simulink model "Array"
settings: Solver=VariableStepDiscrete  StartTime=0.0  StopTime=0.003  RelTol=1e-9  AbsTol=1e-9
values from neighbouring files (symbols this model uses):
  a11 = 300    [matlab1.mat]
  a12 = 200    [matlab1.mat]
  a13 = 100    [matlab1.mat]
  a14 = 100    [matlab1.mat]
  a15 = 100    [matlab1.mat]
  a16 = 100    [matlab1.mat]
  a21 = 200    [matlab1.mat]
  a22 = 100    [matlab1.mat]
  a23 = 100    [matlab1.mat]
  a24 = 1000    [matlab1.mat]
  a25 = 100    [matlab1.mat]
  a26 = 100    [matlab1.mat]
  a31 = 100    [matlab1.mat]
  a32 = 100    [matlab1.mat]
  a33 = 100    [matlab1.mat]
  a34 = 100    [matlab1.mat]
  a35 = 100    [matlab1.mat]
  a36 = 100    [matlab1.mat]
  a41 = 100    [matlab1.mat]
  a42 = 100    [matlab1.mat]
  a43 = 100    [matlab1.mat]
  a44 = 100    [matlab1.mat]
  a45 = 100    [matlab1.mat]
  a46 = 100    [matlab1.mat]
  a51 = 100    [matlab1.mat]
  a52 = 100    [matlab1.mat]
  a53 = 100    [matlab1.mat]
  a54 = 100    [matlab1.mat]
  a55 = 100    [matlab1.mat]
  a56 = 100    [matlab1.mat]
  a61 = 100    [matlab1.mat]
  a62 = 100    [matlab1.mat]
  a63 = 100    [matlab1.mat]
  a64 = 100    [matlab1.mat]
  a65 = 100    [matlab1.mat]
  a66 = 100    [matlab1.mat]
libraries: powerlib x154
(part 2 of 2)

== system Array/Array/PV panel35 ==
  Radiación : Inport
  Temperatura : Inport  Port=2
  Controlled Current Source : powerlib/Electrical Sources/Controlled Current Source  Initialize=on  Source_Type=AC  Amplitude=0  Phase=0  Frequency=0  Measurements=None
  Diode : powerlib/Power Electronics/Diode  Ron=0.001  Lon=0  Vf=0  IC=0  UseSnubber=off  Rs=500  Cs=250e-9  Measurements=off
  PV module : MATLAB Function  TreatAsAtomicUnit=on
  Vpv array : powerlib/Measurements/Voltage Measurement  PhasorSimulation=off  OutputType=Complex  PSBequivalent=0
  + : PMIOPort  Tag=PMCPort  Port=1  Side=Right
  - : PMIOPort  Tag=PMCPort  Port=2  Side=Right
  Ipv : Outport
  Vpv : Outport  Port=2
  wires:
  Radiación/1 -> PV module/2(Radiacion)
  Temperatura/1 -> PV module/3(Temp)
  PV module/1(I) -> Controlled Current Source/1, Ipv/1
  Vpv array/1 -> PV module/1(V), Vpv/1
  connections:
  Controlled Current Source/LConn1 -- Diode/LConn1 -- -/RConn1 -- Vpv array/LConn2
  Controlled Current Source/RConn1 -- Diode/RConn1 -- +/RConn1 -- Vpv array/LConn1

== system Array/Array/PV panel4 ==
  Radiación : Inport
  Temperatura : Inport  Port=2
  Controlled Current Source : powerlib/Electrical Sources/Controlled Current Source  Initialize=on  Source_Type=AC  Amplitude=0  Phase=0  Frequency=0  Measurements=None
  Diode : powerlib/Power Electronics/Diode  Ron=0.001  Lon=0  Vf=0  IC=0  UseSnubber=off  Rs=500  Cs=250e-9  Measurements=off
  PV module : MATLAB Function  TreatAsAtomicUnit=on
  Vpv array : powerlib/Measurements/Voltage Measurement  PhasorSimulation=off  OutputType=Complex  PSBequivalent=0
  + : PMIOPort  Tag=PMCPort  Port=1  Side=Right
  - : PMIOPort  Tag=PMCPort  Port=2  Side=Right
  Ipv : Outport
  Vpv : Outport  Port=2
  wires:
  Radiación/1 -> PV module/2(Radiacion)
  Temperatura/1 -> PV module/3(Temp)
  PV module/1(I) -> Controlled Current Source/1, Ipv/1
  Vpv array/1 -> PV module/1(V), Vpv/1
  connections:
  Controlled Current Source/LConn1 -- Diode/LConn1 -- -/RConn1 -- Vpv array/LConn2
  Controlled Current Source/RConn1 -- Diode/RConn1 -- +/RConn1 -- Vpv array/LConn1

== system Array/Array/PV panel5 ==
  Radiación : Inport
  Temperatura : Inport  Port=2
  Controlled Current Source : powerlib/Electrical Sources/Controlled Current Source  Initialize=on  Source_Type=AC  Amplitude=0  Phase=0  Frequency=0  Measurements=None
  Diode : powerlib/Power Electronics/Diode  Ron=0.001  Lon=0  Vf=0  IC=0  UseSnubber=off  Rs=500  Cs=250e-9  Measurements=off
  PV module : MATLAB Function  TreatAsAtomicUnit=on
  Vpv array : powerlib/Measurements/Voltage Measurement  PhasorSimulation=off  OutputType=Complex  PSBequivalent=0
  + : PMIOPort  Tag=PMCPort  Port=1  Side=Right
  - : PMIOPort  Tag=PMCPort  Port=2  Side=Right
  Ipv : Outport
  Vpv : Outport  Port=2
  wires:
  Radiación/1 -> PV module/2(Radiacion)
  Temperatura/1 -> PV module/3(Temp)
  PV module/1(I) -> Controlled Current Source/1, Ipv/1
  Vpv array/1 -> PV module/1(V), Vpv/1
  connections:
  Controlled Current Source/LConn1 -- Diode/LConn1 -- -/RConn1 -- Vpv array/LConn2
  Controlled Current Source/RConn1 -- Diode/RConn1 -- +/RConn1 -- Vpv array/LConn1

== system Array/Array/PV panel6 ==
  Radiación : Inport
  Temperatura : Inport  Port=2
  Controlled Current Source : powerlib/Electrical Sources/Controlled Current Source  Initialize=on  Source_Type=AC  Amplitude=0  Phase=0  Frequency=0  Measurements=None
  Diode : powerlib/Power Electronics/Diode  Ron=0.001  Lon=0  Vf=0  IC=0  UseSnubber=off  Rs=500  Cs=250e-9  Measurements=off
  PV module : MATLAB Function  TreatAsAtomicUnit=on
  Vpv array : powerlib/Measurements/Voltage Measurement  PhasorSimulation=off  OutputType=Complex  PSBequivalent=0
  + : PMIOPort  Tag=PMCPort  Port=1  Side=Right
  - : PMIOPort  Tag=PMCPort  Port=2  Side=Right
  Ipv : Outport
  Vpv : Outport  Port=2
  wires:
  Radiación/1 -> PV module/2(Radiacion)
  Temperatura/1 -> PV module/3(Temp)
  PV module/1(I) -> Controlled Current Source/1, Ipv/1
  Vpv array/1 -> PV module/1(V), Vpv/1
  connections:
  Controlled Current Source/LConn1 -- Diode/LConn1 -- -/RConn1 -- Vpv array/LConn2
  Controlled Current Source/RConn1 -- Diode/RConn1 -- +/RConn1 -- Vpv array/LConn1

== system Array/Array/PV panel7 ==
  Radiación : Inport
  Temperatura : Inport  Port=2
  Controlled Current Source : powerlib/Electrical Sources/Controlled Current Source  Initialize=on  Source_Type=AC  Amplitude=0  Phase=0  Frequency=0  Measurements=None
  Diode : powerlib/Power Electronics/Diode  Ron=0.001  Lon=0  Vf=0  IC=0  UseSnubber=off  Rs=500  Cs=250e-9  Measurements=off
  PV module : MATLAB Function  TreatAsAtomicUnit=on
  Vpv array : powerlib/Measurements/Voltage Measurement  PhasorSimulation=off  OutputType=Complex  PSBequivalent=0
  + : PMIOPort  Tag=PMCPort  Port=1  Side=Right
  - : PMIOPort  Tag=PMCPort  Port=2  Side=Right
  Ipv : Outport
  Vpv : Outport  Port=2
  wires:
  Radiación/1 -> PV module/2(Radiacion)
  Temperatura/1 -> PV module/3(Temp)
  PV module/1(I) -> Controlled Current Source/1, Ipv/1
  Vpv array/1 -> PV module/1(V), Vpv/1
  connections:
  Controlled Current Source/LConn1 -- Diode/LConn1 -- -/RConn1 -- Vpv array/LConn2
  Controlled Current Source/RConn1 -- Diode/RConn1 -- +/RConn1 -- Vpv array/LConn1

== system Array/Array/PV panel8 ==
  Radiación : Inport
  Temperatura : Inport  Port=2
  Controlled Current Source : powerlib/Electrical Sources/Controlled Current Source  Initialize=on  Source_Type=AC  Amplitude=0  Phase=0  Frequency=0  Measurements=None
  Diode : powerlib/Power Electronics/Diode  Ron=0.001  Lon=0  Vf=0  IC=0  UseSnubber=off  Rs=500  Cs=250e-9  Measurements=off
  PV module : MATLAB Function  TreatAsAtomicUnit=on
  Vpv array : powerlib/Measurements/Voltage Measurement  PhasorSimulation=off  OutputType=Complex  PSBequivalent=0
  + : PMIOPort  Tag=PMCPort  Port=1  Side=Right
  - : PMIOPort  Tag=PMCPort  Port=2  Side=Right
  Ipv : Outport
  Vpv : Outport  Port=2
  wires:
  Radiación/1 -> PV module/2(Radiacion)
  Temperatura/1 -> PV module/3(Temp)
  PV module/1(I) -> Controlled Current Source/1, Ipv/1
  Vpv array/1 -> PV module/1(V), Vpv/1
  connections:
  Controlled Current Source/LConn1 -- Diode/LConn1 -- -/RConn1 -- Vpv array/LConn2
  Controlled Current Source/RConn1 -- Diode/RConn1 -- +/RConn1 -- Vpv array/LConn1

== system Array/Array/PV panel9 ==
  Radiación : Inport
  Temperatura : Inport  Port=2
  Controlled Current Source : powerlib/Electrical Sources/Controlled Current Source  Initialize=on  Source_Type=AC  Amplitude=0  Phase=0  Frequency=0  Measurements=None
  Diode : powerlib/Power Electronics/Diode  Ron=0.001  Lon=0  Vf=0  IC=0  UseSnubber=off  Rs=500  Cs=250e-9  Measurements=off
  PV module : MATLAB Function  TreatAsAtomicUnit=on
  Vpv array : powerlib/Measurements/Voltage Measurement  PhasorSimulation=off  OutputType=Complex  PSBequivalent=0
  + : PMIOPort  Tag=PMCPort  Port=1  Side=Right
  - : PMIOPort  Tag=PMCPort  Port=2  Side=Right
  Ipv : Outport
  Vpv : Outport  Port=2
  wires:
  Radiación/1 -> PV module/2(Radiacion)
  Temperatura/1 -> PV module/3(Temp)
  PV module/1(I) -> Controlled Current Source/1, Ipv/1
  Vpv array/1 -> PV module/1(V), Vpv/1
  connections:
  Controlled Current Source/LConn1 -- Diode/LConn1 -- -/RConn1 -- Vpv array/LConn2
  Controlled Current Source/RConn1 -- Diode/RConn1 -- +/RConn1 -- Vpv array/LConn1

== matlab function Array/PV panel1/PV module ==
  data: V input; I output; Radiacion input; Temp input
function I = Panel (V,Radiacion,Temp)
% Carga del Electron
q=1.602176e-19;
% Contante de Boltzman
K=1.3806488e-23;
% Constante del material
n=1.3;
% Temperatura en Kelvin
T=273.15+Temp;
% Resistencia serie
Rs=0.015;
% Resistencia Paralelo
Rp=100;
% Calculo del producto de constantes de la exponencial
Vt=(n*K*T)/q;
Ns=36; %celdas en serie.
Vc=V./Ns;
% Corriente de Fotogenerada
Isc=5.433;
Alfa=0.037/100;
%variacion de la corriente con la temperatura
Iph=Isc*Radiacion/1000*(1+(Alfa*(Temp-25)));
% Corriente inversa del diodo
Voc_ref=22.2/Ns;
Beta=-0.34/100;
Voc=Voc_ref*(1+(Beta*(Temp-25)));
%for i=1:length(Vc)
%if (Vc(i)>Voc)
%Vc(i)=Voc;
%end
%end
Io=Isc/(exp(Voc/Vt)-1);
Ir=Io;%*(T/298.15)^3*exp(((T/298.15)-1)*1.11*q/(n*K*298.15));

% Funcion a Valuar
I=zeros(size(Vc));
for i=1:50
I = I - (Iph - I - Ir .* ( exp((Vc + I .* Rs) ./ Vt) -1)+(Vc + I .* Rs)/Rp)... 
        ./ (-1 - Ir * (Rs ./ Vt) .* exp((Vc + I .* Rs) ./ Vt)-Rs/Rp); 
end
 end

== matlab function Array/PV panel/PV module ==
  data: V input; I output; Radiacion input; Temp input
function I = Panel (V,Radiacion,Temp)
% Carga del Electron
q=1.602176e-19;
% Contante de Boltzman
K=1.3806488e-23;
% Constante del material
n=1.3;
% Temperatura en Kelvin
T=273.15+Temp;
% Resistencia serie
Rs=0.015;
% Resistencia Paralelo
Rp=100;
% Calculo del producto de constantes de la exponencial
Vt=(n*K*T)/q;
Ns=36; %celdas en serie.
Vc=V./Ns;
% Corriente de Fotogenerada
Isc=5.433;
Alfa=0.037/100;
%variacion de la corriente con la temperatura
Iph=Isc*Radiacion/1000*(1+(Alfa*(Temp-25)));
% Corriente inversa del diodo
Voc_ref=22.2/Ns;
Beta=-0.34/100;
Voc=Voc_ref*(1+(Beta*(Temp-25)));
%for i=1:length(Vc)
%if (Vc(i)>Voc)
%Vc(i)=Voc;
%end
%end
Io=Isc/(exp(Voc/Vt)-1);
Ir=Io;%*(T/298.15)^3*exp(((T/298.15)-1)*1.11*q/(n*K*298.15));

% Funcion a Valuar
I=zeros(size(Vc));
for i=1:50
I = I - (Iph - I - Ir .* ( exp((Vc + I .* Rs) ./ Vt) -1)+(Vc + I .* Rs)/Rp)... 
        ./ (-1 - Ir * (Rs ./ Vt) .* exp((Vc + I .* Rs) ./ Vt)-Rs/Rp); 
end
 end

== matlab function Array/PV panel2/PV module ==
  data: V input; I output; Radiacion input; Temp input
function I = Panel (V,Radiacion,Temp)
% Carga del Electron
q=1.602176e-19;
% Contante de Boltzman
K=1.3806488e-23;
% Constante del material
n=1.3;
% Temperatura en Kelvin
T=273.15+Temp;
% Resistencia serie
Rs=0.015;
% Resistencia Paralelo
Rp=100;
% Calculo del producto de constantes de la exponencial
Vt=(n*K*T)/q;
Ns=36; %celdas en serie.
Vc=V./Ns;
% Corriente de Fotogenerada
Isc=5.433;
Alfa=0.037/100;
%variacion de la corriente con la temperatura
Iph=Isc*Radiacion/1000*(1+(Alfa*(Temp-25)));
% Corriente inversa del diodo
Voc_ref=22.2/Ns;
Beta=-0.34/100;
Voc=Voc_ref*(1+(Beta*(Temp-25)));
%for i=1:length(Vc)
%if (Vc(i)>Voc)
%Vc(i)=Voc;
%end
%end
Io=Isc/(exp(Voc/Vt)-1);
Ir=Io;%*(T/298.15)^3*exp(((T/298.15)-1)*1.11*q/(n*K*298.15));

% Funcion a Valuar
I=zeros(size(Vc));
for i=1:50
I = I - (Iph - I - Ir .* ( exp((Vc + I .* Rs) ./ Vt) -1)+(Vc + I .* Rs)/Rp)... 
        ./ (-1 - Ir * (Rs ./ Vt) .* exp((Vc + I .* Rs) ./ Vt)-Rs/Rp); 
end
 end

== matlab function Array/PV panel3/PV module ==
  data: V input; I output; Radiacion input; Temp input
function I = Panel (V,Radiacion,Temp)
% Carga del Electron
q=1.602176e-19;
% Contante de Boltzman
K=1.3806488e-23;
% Constante del material
n=1.3;
% Temperatura en Kelvin
T=273.15+Temp;
% Resistencia serie
Rs=0.015;
% Resistencia Paralelo
Rp=100;
% Calculo del producto de constantes de la exponencial
Vt=(n*K*T)/q;
Ns=36; %celdas en serie.
Vc=V./Ns;
% Corriente de Fotogenerada
Isc=5.433;
Alfa=0.037/100;
%variacion de la corriente con la temperatura
Iph=Isc*Radiacion/1000*(1+(Alfa*(Temp-25)));
% Corriente inversa del diodo
Voc_ref=22.2/Ns;
Beta=-0.34/100;
Voc=Voc_ref*(1+(Beta*(Temp-25)));
%for i=1:length(Vc)
%if (Vc(i)>Voc)
%Vc(i)=Voc;
%end
%end
Io=Isc/(exp(Voc/Vt)-1);
Ir=Io;%*(T/298.15)^3*exp(((T/298.15)-1)*1.11*q/(n*K*298.15));

% Funcion a Valuar
I=zeros(size(Vc));
for i=1:50
I = I - (Iph - I - Ir .* ( exp((Vc + I .* Rs) ./ Vt) -1)+(Vc + I .* Rs)/Rp)... 
        ./ (-1 - Ir * (Rs ./ Vt) .* exp((Vc + I .* Rs) ./ Vt)-Rs/Rp); 
end
 end

== matlab function Array/PV panel4/PV module ==
  data: V input; I output; Radiacion input; Temp input
function I = Panel (V,Radiacion,Temp)
% Carga del Electron
q=1.602176e-19;
% Contante de Boltzman
K=1.3806488e-23;
% Constante del material
n=1.3;
% Temperatura en Kelvin
T=273.15+Temp;
% Resistencia serie
Rs=0.015;
% Resistencia Paralelo
Rp=100;
% Calculo del producto de constantes de la exponencial
Vt=(n*K*T)/q;
Ns=36; %celdas en serie.
Vc=V./Ns;
% Corriente de Fotogenerada
Isc=5.433;
Alfa=0.037/100;
%variacion de la corriente con la temperatura
Iph=Isc*Radiacion/1000*(1+(Alfa*(Temp-25)));
% Corriente inversa del diodo
Voc_ref=22.2/Ns;
Beta=-0.34/100;
Voc=Voc_ref*(1+(Beta*(Temp-25)));
%for i=1:length(Vc)
%if (Vc(i)>Voc)
%Vc(i)=Voc;
%end
%end
Io=Isc/(exp(Voc/Vt)-1);
Ir=Io;%*(T/298.15)^3*exp(((T/298.15)-1)*1.11*q/(n*K*298.15));

% Funcion a Valuar
I=zeros(size(Vc));
for i=1:50
I = I - (Iph - I - Ir .* ( exp((Vc + I .* Rs) ./ Vt) -1)+(Vc + I .* Rs)/Rp)... 
        ./ (-1 - Ir * (Rs ./ Vt) .* exp((Vc + I .* Rs) ./ Vt)-Rs/Rp); 
end
 end

== matlab function Array/PV panel5/PV module ==
  data: V input; I output; Radiacion input; Temp input
function I = Panel (V,Radiacion,Temp)
% Carga del Electron
q=1.602176e-19;
% Contante de Boltzman
K=1.3806488e-23;
% Constante del material
n=1.3;
% Temperatura en Kelvin
T=273.15+Temp;
% Resistencia serie
Rs=0.015;
% Resistencia Paralelo
Rp=100;
% Calculo del producto de constantes de la exponencial
Vt=(n*K*T)/q;
Ns=36; %celdas en serie.
Vc=V./Ns;
% Corriente de Fotogenerada
Isc=5.433;
Alfa=0.037/100;
%variacion de la corriente con la temperatura
Iph=Isc*Radiacion/1000*(1+(Alfa*(Temp-25)));
% Corriente inversa del diodo
Voc_ref=22.2/Ns;
Beta=-0.34/100;
Voc=Voc_ref*(1+(Beta*(Temp-25)));
%for i=1:length(Vc)
%if (Vc(i)>Voc)
%Vc(i)=Voc;
%end
%end
Io=Isc/(exp(Voc/Vt)-1);
Ir=Io;%*(T/298.15)^3*exp(((T/298.15)-1)*1.11*q/(n*K*298.15));

% Funcion a Valuar
I=zeros(size(Vc));
for i=1:50
I = I - (Iph - I - Ir .* ( exp((Vc + I .* Rs) ./ Vt) -1)+(Vc + I .* Rs)/Rp)... 
        ./ (-1 - Ir * (Rs ./ Vt) .* exp((Vc + I .* Rs) ./ Vt)-Rs/Rp); 
end
 end

== matlab function Array/PV panel6/PV module ==
  data: V input; I output; Radiacion input; Temp input
function I = Panel (V,Radiacion,Temp)
% Carga del Electron
q=1.602176e-19;
% Contante de Boltzman
K=1.3806488e-23;
% Constante del material
n=1.3;
% Temperatura en Kelvin
T=273.15+Temp;
% Resistencia serie
Rs=0.015;
% Resistencia Paralelo
Rp=100;
% Calculo del producto de constantes de la exponencial
Vt=(n*K*T)/q;
Ns=36; %celdas en serie.
Vc=V./Ns;
% Corriente de Fotogenerada
Isc=5.433;
Alfa=0.037/100;
%variacion de la corriente con la temperatura
Iph=Isc*Radiacion/1000*(1+(Alfa*(Temp-25)));
% Corriente inversa del diodo
Voc_ref=22.2/Ns;
Beta=-0.34/100;
Voc=Voc_ref*(1+(Beta*(Temp-25)));
%for i=1:length(Vc)
%if (Vc(i)>Voc)
%Vc(i)=Voc;
%end
%end
Io=Isc/(exp(Voc/Vt)-1);
Ir=Io;%*(T/298.15)^3*exp(((T/298.15)-1)*1.11*q/(n*K*298.15));

% Funcion a Valuar
I=zeros(size(Vc));
for i=1:50
I = I - (Iph - I - Ir .* ( exp((Vc + I .* Rs) ./ Vt) -1)+(Vc + I .* Rs)/Rp)... 
        ./ (-1 - Ir * (Rs ./ Vt) .* exp((Vc + I .* Rs) ./ Vt)-Rs/Rp); 
end
 end

== matlab function Array/PV panel7/PV module ==
  data: V input; I output; Radiacion input; Temp input
function I = Panel (V,Radiacion,Temp)
% Carga del Electron
q=1.602176e-19;
% Contante de Boltzman
K=1.3806488e-23;
% Constante del material
n=1.3;
% Temperatura en Kelvin
T=273.15+Temp;
% Resistencia serie
Rs=0.015;
% Resistencia Paralelo
Rp=100;
% Calculo del producto de constantes de la exponencial
Vt=(n*K*T)/q;
Ns=36; %celdas en serie.
Vc=V./Ns;
% Corriente de Fotogenerada
Isc=5.433;
Alfa=0.037/100;
%variacion de la corriente con la temperatura
Iph=Isc*Radiacion/1000*(1+(Alfa*(Temp-25)));
% Corriente inversa del diodo
Voc_ref=22.2/Ns;
Beta=-0.34/100;
Voc=Voc_ref*(1+(Beta*(Temp-25)));
%for i=1:length(Vc)
%if (Vc(i)>Voc)
%Vc(i)=Voc;
%end
%end
Io=Isc/(exp(Voc/Vt)-1);
Ir=Io;%*(T/298.15)^3*exp(((T/298.15)-1)*1.11*q/(n*K*298.15));

% Funcion a Valuar
I=zeros(size(Vc));
for i=1:50
I = I - (Iph - I - Ir .* ( exp((Vc + I .* Rs) ./ Vt) -1)+(Vc + I .* Rs)/Rp)... 
        ./ (-1 - Ir * (Rs ./ Vt) .* exp((Vc + I .* Rs) ./ Vt)-Rs/Rp); 
end
 end

== matlab function Array/PV panel8/PV module ==
  data: V input; I output; Radiacion input; Temp input
function I = Panel (V,Radiacion,Temp)
% Carga del Electron
q=1.602176e-19;
% Contante de Boltzman
K=1.3806488e-23;
% Constante del material
n=1.3;
% Temperatura en Kelvin
T=273.15+Temp;
% Resistencia serie
Rs=0.015;
% Resistencia Paralelo
Rp=100;
% Calculo del producto de constantes de la exponencial
Vt=(n*K*T)/q;
Ns=36; %celdas en serie.
Vc=V./Ns;
% Corriente de Fotogenerada
Isc=5.433;
Alfa=0.037/100;
%variacion de la corriente con la temperatura
Iph=Isc*Radiacion/1000*(1+(Alfa*(Temp-25)));
% Corriente inversa del diodo
Voc_ref=22.2/Ns;
Beta=-0.34/100;
Voc=Voc_ref*(1+(Beta*(Temp-25)));
%for i=1:length(Vc)
%if (Vc(i)>Voc)
%Vc(i)=Voc;
%end
%end
Io=Isc/(exp(Voc/Vt)-1);
Ir=Io;%*(T/298.15)^3*exp(((T/298.15)-1)*1.11*q/(n*K*298.15));

% Funcion a Valuar
I=zeros(size(Vc));
for i=1:50
I = I - (Iph - I - Ir .* ( exp((Vc + I .* Rs) ./ Vt) -1)+(Vc + I .* Rs)/Rp)... 
        ./ (-1 - Ir * (Rs ./ Vt) .* exp((Vc + I .* Rs) ./ Vt)-Rs/Rp); 
end
 end

== matlab function Array/PV panel10/PV module ==
  data: V input; I output; Radiacion input; Temp input
function I = Panel (V,Radiacion,Temp)
% Carga del Electron
q=1.602176e-19;
% Contante de Boltzman
K=1.3806488e-23;
% Constante del material
n=1.3;
% Temperatura en Kelvin
T=273.15+Temp;
% Resistencia serie
Rs=0.015;
% Resistencia Paralelo
Rp=100;
% Calculo del producto de constantes de la exponencial
Vt=(n*K*T)/q;
Ns=36; %celdas en serie.
Vc=V./Ns;
% Corriente de Fotogenerada
Isc=5.433;
Alfa=0.037/100;
%variacion de la corriente con la temperatura
Iph=Isc*Radiacion/1000*(1+(Alfa*(Temp-25)));
% Corriente inversa del diodo
Voc_ref=22.2/Ns;
Beta=-0.34/100;
Voc=Voc_ref*(1+(Beta*(Temp-25)));
%for i=1:length(Vc)
%if (Vc(i)>Voc)
%Vc(i)=Voc;
%end
%end
Io=Isc/(exp(Voc/Vt)-1);
Ir=Io;%*(T/298.15)^3*exp(((T/298.15)-1)*1.11*q/(n*K*298.15));

% Funcion a Valuar
I=zeros(size(Vc));
for i=1:50
I = I - (Iph - I - Ir .* ( exp((Vc + I .* Rs) ./ Vt) -1)+(Vc + I .* Rs)/Rp)... 
        ./ (-1 - Ir * (Rs ./ Vt) .* exp((Vc + I .* Rs) ./ Vt)-Rs/Rp); 
end
 end

== matlab function Array/PV panel11/PV module ==
  data: V input; I output; Radiacion input; Temp input
function I = Panel (V,Radiacion,Temp)
% Carga del Electron
q=1.602176e-19;
% Contante de Boltzman
K=1.3806488e-23;
% Constante del material
n=1.3;
% Temperatura en Kelvin
T=273.15+Temp;
% Resistencia serie
Rs=0.015;
% Resistencia Paralelo
Rp=100;
% Calculo del producto de constantes de la exponencial
Vt=(n*K*T)/q;
Ns=36; %celdas en serie.
Vc=V./Ns;
% Corriente de Fotogenerada
Isc=5.433;
Alfa=0.037/100;
%variacion de la corriente con la temperatura
Iph=Isc*Radiacion/1000*(1+(Alfa*(Temp-25)));
% Corriente inversa del diodo
Voc_ref=22.2/Ns;
Beta=-0.34/100;
Voc=Voc_ref*(1+(Beta*(Temp-25)));
%for i=1:length(Vc)
%if (Vc(i)>Voc)
%Vc(i)=Voc;
%end
%end
Io=Isc/(exp(Voc/Vt)-1);
Ir=Io;%*(T/298.15)^3*exp(((T/298.15)-1)*1.11*q/(n*K*298.15));

% Funcion a Valuar
I=zeros(size(Vc));
for i=1:50
I = I - (Iph - I - Ir .* ( exp((Vc + I .* Rs) ./ Vt) -1)+(Vc + I .* Rs)/Rp)... 
        ./ (-1 - Ir * (Rs ./ Vt) .* exp((Vc + I .* Rs) ./ Vt)-Rs/Rp); 
end
 end

== matlab function Array/PV panel12/PV module ==
  data: V input; I output; Radiacion input; Temp input
function I = Panel (V,Radiacion,Temp)
% Carga del Electron
q=1.602176e-19;
% Contante de Boltzman
K=1.3806488e-23;
% Constante del material
n=1.3;
% Temperatura en Kelvin
T=273.15+Temp;
% Resistencia serie
Rs=0.015;
% Resistencia Paralelo
Rp=100;
% Calculo del producto de constantes de la exponencial
Vt=(n*K*T)/q;
Ns=36; %celdas en serie.
Vc=V./Ns;
% Corriente de Fotogenerada
Isc=5.433;
Alfa=0.037/100;
%variacion de la corriente con la temperatura
Iph=Isc*Radiacion/1000*(1+(Alfa*(Temp-25)));
% Corriente inversa del diodo
Voc_ref=22.2/Ns;
Beta=-0.34/100;
Voc=Voc_ref*(1+(Beta*(Temp-25)));
%for i=1:length(Vc)
%if (Vc(i)>Voc)
%Vc(i)=Voc;
%end
%end
Io=Isc/(exp(Voc/Vt)-1);
Ir=Io;%*(T/298.15)^3*exp(((T/298.15)-1)*1.11*q/(n*K*298.15));

% Funcion a Valuar
I=zeros(size(Vc));
for i=1:50
I = I - (Iph - I - Ir .* ( exp((Vc + I .* Rs) ./ Vt) -1)+(Vc + I .* Rs)/Rp)... 
        ./ (-1 - Ir * (Rs ./ Vt) .* exp((Vc + I .* Rs) ./ Vt)-Rs/Rp); 
end
 end

== matlab function Array/PV panel13/PV module ==
  data: V input; I output; Radiacion input; Temp input
function I = Panel (V,Radiacion,Temp)
% Carga del Electron
q=1.602176e-19;
% Contante de Boltzman
K=1.3806488e-23;
% Constante del material
n=1.3;
% Temperatura en Kelvin
T=273.15+Temp;
% Resistencia serie
Rs=0.015;
% Resistencia Paralelo
Rp=100;
% Calculo del producto de constantes de la exponencial
Vt=(n*K*T)/q;
Ns=36; %celdas en serie.
Vc=V./Ns;
% Corriente de Fotogenerada
Isc=5.433;
Alfa=0.037/100;
%variacion de la corriente con la temperatura
Iph=Isc*Radiacion/1000*(1+(Alfa*(Temp-25)));
% Corriente inversa del diodo
Voc_ref=22.2/Ns;
Beta=-0.34/100;
Voc=Voc_ref*(1+(Beta*(Temp-25)));
%for i=1:length(Vc)
%if (Vc(i)>Voc)
%Vc(i)=Voc;
%end
%end
Io=Isc/(exp(Voc/Vt)-1);
Ir=Io;%*(T/298.15)^3*exp(((T/298.15)-1)*1.11*q/(n*K*298.15));

% Funcion a Valuar
I=zeros(size(Vc));
for i=1:50
I = I - (Iph - I - Ir .* ( exp((Vc + I .* Rs) ./ Vt) -1)+(Vc + I .* Rs)/Rp)... 
        ./ (-1 - Ir * (Rs ./ Vt) .* exp((Vc + I .* Rs) ./ Vt)-Rs/Rp); 
end
 end

== matlab function Array/PV panel14/PV module ==
  data: V input; I output; Radiacion input; Temp input
function I = Panel (V,Radiacion,Temp)
% Carga del Electron
q=1.602176e-19;
% Contante de Boltzman
K=1.3806488e-23;
% Constante del material
n=1.3;
% Temperatura en Kelvin
T=273.15+Temp;
% Resistencia serie
Rs=0.015;
% Resistencia Paralelo
Rp=100;
% Calculo del producto de constantes de la exponencial
Vt=(n*K*T)/q;
Ns=36; %celdas en serie.
Vc=V./Ns;
% Corriente de Fotogenerada
Isc=5.433;
Alfa=0.037/100;
%variacion de la corriente con la temperatura
Iph=Isc*Radiacion/1000*(1+(Alfa*(Temp-25)));
% Corriente inversa del diodo
Voc_ref=22.2/Ns;
Beta=-0.34/100;
Voc=Voc_ref*(1+(Beta*(Temp-25)));
%for i=1:length(Vc)
%if (Vc(i)>Voc)
%Vc(i)=Voc;
%end
%end
Io=Isc/(exp(Voc/Vt)-1);
Ir=Io;%*(T/298.15)^3*exp(((T/298.15)-1)*1.11*q/(n*K*298.15));

% Funcion a Valuar
I=zeros(size(Vc));
for i=1:50
I = I - (Iph - I - Ir .* ( exp((Vc + I .* Rs) ./ Vt) -1)+(Vc + I .* Rs)/Rp)... 
        ./ (-1 - Ir * (Rs ./ Vt) .* exp((Vc + I .* Rs) ./ Vt)-Rs/Rp); 
end
 end

== matlab function Array/PV panel15/PV module ==
  data: V input; I output; Radiacion input; Temp input
function I = Panel (V,Radiacion,Temp)
% Carga del Electron
q=1.602176e-19;
% Contante de Boltzman
K=1.3806488e-23;
% Constante del material
n=1.3;
% Temperatura en Kelvin
T=273.15+Temp;
% Resistencia serie
Rs=0.015;
% Resistencia Paralelo
Rp=100;
% Calculo del producto de constantes de la exponencial
Vt=(n*K*T)/q;
Ns=36; %celdas en serie.
Vc=V./Ns;
% Corriente de Fotogenerada
Isc=5.433;
Alfa=0.037/100;
%variacion de la corriente con la temperatura
Iph=Isc*Radiacion/1000*(1+(Alfa*(Temp-25)));
% Corriente inversa del diodo
Voc_ref=22.2/Ns;
Beta=-0.34/100;
Voc=Voc_ref*(1+(Beta*(Temp-25)));
%for i=1:length(Vc)
%if (Vc(i)>Voc)
%Vc(i)=Voc;
%end
%end
Io=Isc/(exp(Voc/Vt)-1);
Ir=Io;%*(T/298.15)^3*exp(((T/298.15)-1)*1.11*q/(n*K*298.15));

% Funcion a Valuar
I=zeros(size(Vc));
for i=1:50
I = I - (Iph - I - Ir .* ( exp((Vc + I .* Rs) ./ Vt) -1)+(Vc + I .* Rs)/Rp)... 
        ./ (-1 - Ir * (Rs ./ Vt) .* exp((Vc + I .* Rs) ./ Vt)-Rs/Rp); 
end
 end

== matlab function Array/PV panel16/PV module ==
  data: V input; I output; Radiacion input; Temp input
function I = Panel (V,Radiacion,Temp)
% Carga del Electron
q=1.602176e-19;
% Contante de Boltzman
K=1.3806488e-23;
% Constante del material
n=1.3;
% Temperatura en Kelvin
T=273.15+Temp;
% Resistencia serie
Rs=0.015;
% Resistencia Paralelo
Rp=100;
% Calculo del producto de constantes de la exponencial
Vt=(n*K*T)/q;
Ns=36; %celdas en serie.
Vc=V./Ns;
% Corriente de Fotogenerada
Isc=5.433;
Alfa=0.037/100;
%variacion de la corriente con la temperatura
Iph=Isc*Radiacion/1000*(1+(Alfa*(Temp-25)));
% Corriente inversa del diodo
Voc_ref=22.2/Ns;
Beta=-0.34/100;
Voc=Voc_ref*(1+(Beta*(Temp-25)));
%for i=1:length(Vc)
%if (Vc(i)>Voc)
%Vc(i)=Voc;
%end
%end
Io=Isc/(exp(Voc/Vt)-1);
Ir=Io;%*(T/298.15)^3*exp(((T/298.15)-1)*1.11*q/(n*K*298.15));

% Funcion a Valuar
I=zeros(size(Vc));
for i=1:50
I = I - (Iph - I - Ir .* ( exp((Vc + I .* Rs) ./ Vt) -1)+(Vc + I .* Rs)/Rp)... 
        ./ (-1 - Ir * (Rs ./ Vt) .* exp((Vc + I .* Rs) ./ Vt)-Rs/Rp); 
end
 end

== matlab function Array/PV panel17/PV module ==
  data: V input; I output; Radiacion input; Temp input
function I = Panel (V,Radiacion,Temp)
% Carga del Electron
q=1.602176e-19;
% Contante de Boltzman
K=1.3806488e-23;
% Constante del material
n=1.3;
% Temperatura en Kelvin
T=273.15+Temp;
% Resistencia serie
Rs=0.015;
% Resistencia Paralelo
Rp=100;
% Calculo del producto de constantes de la exponencial
Vt=(n*K*T)/q;
Ns=36; %celdas en serie.
Vc=V./Ns;
% Corriente de Fotogenerada
Isc=5.433;
Alfa=0.037/100;
%variacion de la corriente con la temperatura
Iph=Isc*Radiacion/1000*(1+(Alfa*(Temp-25)));
% Corriente inversa del diodo
Voc_ref=22.2/Ns;
Beta=-0.34/100;
Voc=Voc_ref*(1+(Beta*(Temp-25)));
%for i=1:length(Vc)
%if (Vc(i)>Voc)
%Vc(i)=Voc;
%end
%end
Io=Isc/(exp(Voc/Vt)-1);
Ir=Io;%*(T/298.15)^3*exp(((T/298.15)-1)*1.11*q/(n*K*298.15));

% Funcion a Valuar
I=zeros(size(Vc));
for i=1:50
I = I - (Iph - I - Ir .* ( exp((Vc + I .* Rs) ./ Vt) -1)+(Vc + I .* Rs)/Rp)... 
        ./ (-1 - Ir * (Rs ./ Vt) .* exp((Vc + I .* Rs) ./ Vt)-Rs/Rp); 
end
 end

== matlab function Array/PV panel9/PV module ==
  data: V input; I output; Radiacion input; Temp input
function I = Panel (V,Radiacion,Temp)
% Carga del Electron
q=1.602176e-19;
% Contante de Boltzman
K=1.3806488e-23;
% Constante del material
n=1.3;
% Temperatura en Kelvin
T=273.15+Temp;
% Resistencia serie
Rs=0.015;
% Resistencia Paralelo
Rp=100;
% Calculo del producto de constantes de la exponencial
Vt=(n*K*T)/q;
Ns=36; %celdas en serie.
Vc=V./Ns;
% Corriente de Fotogenerada
Isc=5.433;
Alfa=0.037/100;
%variacion de la corriente con la temperatura
Iph=Isc*Radiacion/1000*(1+(Alfa*(Temp-25)));
% Corriente inversa del diodo
Voc_ref=22.2/Ns;
Beta=-0.34/100;
Voc=Voc_ref*(1+(Beta*(Temp-25)));
%for i=1:length(Vc)
%if (Vc(i)>Voc)
%Vc(i)=Voc;
%end
%end
Io=Isc/(exp(Voc/Vt)-1);
Ir=Io;%*(T/298.15)^3*exp(((T/298.15)-1)*1.11*q/(n*K*298.15));

% Funcion a Valuar
I=zeros(size(Vc));
for i=1:50
I = I - (Iph - I - Ir .* ( exp((Vc + I .* Rs) ./ Vt) -1)+(Vc + I .* Rs)/Rp)... 
        ./ (-1 - Ir * (Rs ./ Vt) .* exp((Vc + I .* Rs) ./ Vt)-Rs/Rp); 
end
 end

== matlab function Array/PV panel18/PV module ==
  data: V input; I output; Radiacion input; Temp input
function I = Panel (V,Radiacion,Temp)
% Carga del Electron
q=1.602176e-19;
% Contante de Boltzman
K=1.3806488e-23;
% Constante del material
n=1.3;
% Temperatura en Kelvin
T=273.15+Temp;
% Resistencia serie
Rs=0.015;
% Resistencia Paralelo
Rp=100;
% Calculo del producto de constantes de la exponencial
Vt=(n*K*T)/q;
Ns=36; %celdas en serie.
Vc=V./Ns;
% Corriente de Fotogenerada
Isc=5.433;
Alfa=0.037/100;
%variacion de la corriente con la temperatura
Iph=Isc*Radiacion/1000*(1+(Alfa*(Temp-25)));
% Corriente inversa del diodo
Voc_ref=22.2/Ns;
Beta=-0.34/100;
Voc=Voc_ref*(1+(Beta*(Temp-25)));
%for i=1:length(Vc)
%if (Vc(i)>Voc)
%Vc(i)=Voc;
%end
%end
Io=Isc/(exp(Voc/Vt)-1);
Ir=Io;%*(T/298.15)^3*exp(((T/298.15)-1)*1.11*q/(n*K*298.15));

% Funcion a Valuar
I=zeros(size(Vc));
for i=1:50
I = I - (Iph - I - Ir .* ( exp((Vc + I .* Rs) ./ Vt) -1)+(Vc + I .* Rs)/Rp)... 
        ./ (-1 - Ir * (Rs ./ Vt) .* exp((Vc + I .* Rs) ./ Vt)-Rs/Rp); 
end
 end

== matlab function Array/PV panel19/PV module ==
  data: V input; I output; Radiacion input; Temp input
function I = Panel (V,Radiacion,Temp)
% Carga del Electron
q=1.602176e-19;
% Contante de Boltzman
K=1.3806488e-23;
% Constante del material
n=1.3;
% Temperatura en Kelvin
T=273.15+Temp;
% Resistencia serie
Rs=0.015;
% Resistencia Paralelo
Rp=100;
% Calculo del producto de constantes de la exponencial
Vt=(n*K*T)/q;
Ns=36; %celdas en serie.
Vc=V./Ns;
% Corriente de Fotogenerada
Isc=5.433;
Alfa=0.037/100;
%variacion de la corriente con la temperatura
Iph=Isc*Radiacion/1000*(1+(Alfa*(Temp-25)));
% Corriente inversa del diodo
Voc_ref=22.2/Ns;
Beta=-0.34/100;
Voc=Voc_ref*(1+(Beta*(Temp-25)));
%for i=1:length(Vc)
%if (Vc(i)>Voc)
%Vc(i)=Voc;
%end
%end
Io=Isc/(exp(Voc/Vt)-1);
Ir=Io;%*(T/298.15)^3*exp(((T/298.15)-1)*1.11*q/(n*K*298.15));

% Funcion a Valuar
I=zeros(size(Vc));
for i=1:50
I = I - (Iph - I - Ir .* ( exp((Vc + I .* Rs) ./ Vt) -1)+(Vc + I .* Rs)/Rp)... 
        ./ (-1 - Ir * (Rs ./ Vt) .* exp((Vc + I .* Rs) ./ Vt)-Rs/Rp); 
end
 end

== matlab function Array/PV panel20/PV module ==
  data: V input; I output; Radiacion input; Temp input
function I = Panel (V,Radiacion,Temp)
% Carga del Electron
q=1.602176e-19;
% Contante de Boltzman
K=1.3806488e-23;
% Constante del material
n=1.3;
% Temperatura en Kelvin
T=273.15+Temp;
% Resistencia serie
Rs=0.015;
% Resistencia Paralelo
Rp=100;
% Calculo del producto de constantes de la exponencial
Vt=(n*K*T)/q;
Ns=36; %celdas en serie.
Vc=V./Ns;
% Corriente de Fotogenerada
Isc=5.433;
Alfa=0.037/100;
%variacion de la corriente con la temperatura
Iph=Isc*Radiacion/1000*(1+(Alfa*(Temp-25)));
% Corriente inversa del diodo
Voc_ref=22.2/Ns;
Beta=-0.34/100;
Voc=Voc_ref*(1+(Beta*(Temp-25)));
%for i=1:length(Vc)
%if (Vc(i)>Voc)
%Vc(i)=Voc;
%end
%end
Io=Isc/(exp(Voc/Vt)-1);
Ir=Io;%*(T/298.15)^3*exp(((T/298.15)-1)*1.11*q/(n*K*298.15));

% Funcion a Valuar
I=zeros(size(Vc));
for i=1:50
I = I - (Iph - I - Ir .* ( exp((Vc + I .* Rs) ./ Vt) -1)+(Vc + I .* Rs)/Rp)... 
        ./ (-1 - Ir * (Rs ./ Vt) .* exp((Vc + I .* Rs) ./ Vt)-Rs/Rp); 
end
 end

== matlab function Array/PV panel21/PV module ==
  data: V input; I output; Radiacion input; Temp input
function I = Panel (V,Radiacion,Temp)
% Carga del Electron
q=1.602176e-19;
% Contante de Boltzman
K=1.3806488e-23;
% Constante del material
n=1.3;
% Temperatura en Kelvin
T=273.15+Temp;
% Resistencia serie
Rs=0.015;
% Resistencia Paralelo
Rp=100;
% Calculo del producto de constantes de la exponencial
Vt=(n*K*T)/q;
Ns=36; %celdas en serie.
Vc=V./Ns;
% Corriente de Fotogenerada
Isc=5.433;
Alfa=0.037/100;
%variacion de la corriente con la temperatura
Iph=Isc*Radiacion/1000*(1+(Alfa*(Temp-25)));
% Corriente inversa del diodo
Voc_ref=22.2/Ns;
Beta=-0.34/100;
Voc=Voc_ref*(1+(Beta*(Temp-25)));
%for i=1:length(Vc)
%if (Vc(i)>Voc)
%Vc(i)=Voc;
%end
%end
Io=Isc/(exp(Voc/Vt)-1);
Ir=Io;%*(T/298.15)^3*exp(((T/298.15)-1)*1.11*q/(n*K*298.15));

% Funcion a Valuar
I=zeros(size(Vc));
for i=1:50
I = I - (Iph - I - Ir .* ( exp((Vc + I .* Rs) ./ Vt) -1)+(Vc + I .* Rs)/Rp)... 
        ./ (-1 - Ir * (Rs ./ Vt) .* exp((Vc + I .* Rs) ./ Vt)-Rs/Rp); 
end
 end

== matlab function Array/PV panel22/PV module ==
  data: V input; I output; Radiacion input; Temp input
function I = Panel (V,Radiacion,Temp)
% Carga del Electron
q=1.602176e-19;
% Contante de Boltzman
K=1.3806488e-23;
% Constante del material
n=1.3;
% Temperatura en Kelvin
T=273.15+Temp;
% Resistencia serie
Rs=0.015;
% Resistencia Paralelo
Rp=100;
% Calculo del producto de constantes de la exponencial
Vt=(n*K*T)/q;
Ns=36; %celdas en serie.
Vc=V./Ns;
% Corriente de Fotogenerada
Isc=5.433;
Alfa=0.037/100;
%variacion de la corriente con la temperatura
Iph=Isc*Radiacion/1000*(1+(Alfa*(Temp-25)));
% Corriente inversa del diodo
Voc_ref=22.2/Ns;
Beta=-0.34/100;
Voc=Voc_ref*(1+(Beta*(Temp-25)));
%for i=1:length(Vc)
%if (Vc(i)>Voc)
%Vc(i)=Voc;
%end
%end
Io=Isc/(exp(Voc/Vt)-1);
Ir=Io;%*(T/298.15)^3*exp(((T/298.15)-1)*1.11*q/(n*K*298.15));

% Funcion a Valuar
I=zeros(size(Vc));
for i=1:50
I = I - (Iph - I - Ir .* ( exp((Vc + I .* Rs) ./ Vt) -1)+(Vc + I .* Rs)/Rp)... 
        ./ (-1 - Ir * (Rs ./ Vt) .* exp((Vc + I .* Rs) ./ Vt)-Rs/Rp); 
end
 end

== matlab function Array/PV panel23/PV module ==
  data: V input; I output; Radiacion input; Temp input
function I = Panel (V,Radiacion,Temp)
% Carga del Electron
q=1.602176e-19;
% Contante de Boltzman
K=1.3806488e-23;
% Constante del material
n=1.3;
% Temperatura en Kelvin
T=273.15+Temp;
% Resistencia serie
Rs=0.015;
% Resistencia Paralelo
Rp=100;
% Calculo del producto de constantes de la exponencial
Vt=(n*K*T)/q;
Ns=36; %celdas en serie.
Vc=V./Ns;
% Corriente de Fotogenerada
Isc=5.433;
Alfa=0.037/100;
%variacion de la corriente con la temperatura
Iph=Isc*Radiacion/1000*(1+(Alfa*(Temp-25)));
% Corriente inversa del diodo
Voc_ref=22.2/Ns;
Beta=-0.34/100;
Voc=Voc_ref*(1+(Beta*(Temp-25)));
%for i=1:length(Vc)
%if (Vc(i)>Voc)
%Vc(i)=Voc;
%end
%end
Io=Isc/(exp(Voc/Vt)-1);
Ir=Io;%*(T/298.15)^3*exp(((T/298.15)-1)*1.11*q/(n*K*298.15));

% Funcion a Valuar
I=zeros(size(Vc));
for i=1:50
I = I - (Iph - I - Ir .* ( exp((Vc + I .* Rs) ./ Vt) -1)+(Vc + I .* Rs)/Rp)... 
        ./ (-1 - Ir * (Rs ./ Vt) .* exp((Vc + I .* Rs) ./ Vt)-Rs/Rp); 
end
 end

== matlab function Array/PV panel24/PV module ==
  data: V input; I output; Radiacion input; Temp input
function I = Panel (V,Radiacion,Temp)
% Carga del Electron
q=1.602176e-19;
% Contante de Boltzman
K=1.3806488e-23;
% Constante del material
n=1.3;
% Temperatura en Kelvin
T=273.15+Temp;
% Resistencia serie
Rs=0.015;
% Resistencia Paralelo
Rp=100;
% Calculo del producto de constantes de la exponencial
Vt=(n*K*T)/q;
Ns=36; %celdas en serie.
Vc=V./Ns;
% Corriente de Fotogenerada
Isc=5.433;
Alfa=0.037/100;
%variacion de la corriente con la temperatura
Iph=Isc*Radiacion/1000*(1+(Alfa*(Temp-25)));
% Corriente inversa del diodo
Voc_ref=22.2/Ns;
Beta=-0.34/100;
Voc=Voc_ref*(1+(Beta*(Temp-25)));
%for i=1:length(Vc)
%if (Vc(i)>Voc)
%Vc(i)=Voc;
%end
%end
Io=Isc/(exp(Voc/Vt)-1);
Ir=Io;%*(T/298.15)^3*exp(((T/298.15)-1)*1.11*q/(n*K*298.15));

% Funcion a Valuar
I=zeros(size(Vc));
for i=1:50
I = I - (Iph - I - Ir .* ( exp((Vc + I .* Rs) ./ Vt) -1)+(Vc + I .* Rs)/Rp)... 
        ./ (-1 - Ir * (Rs ./ Vt) .* exp((Vc + I .* Rs) ./ Vt)-Rs/Rp); 
end
 end

== matlab function Array/PV panel25/PV module ==
  data: V input; I output; Radiacion input; Temp input
function I = Panel (V,Radiacion,Temp)
% Carga del Electron
q=1.602176e-19;
% Contante de Boltzman
K=1.3806488e-23;
% Constante del material
n=1.3;
% Temperatura en Kelvin
T=273.15+Temp;
% Resistencia serie
Rs=0.015;
% Resistencia Paralelo
Rp=100;
% Calculo del producto de constantes de la exponencial
Vt=(n*K*T)/q;
Ns=36; %celdas en serie.
Vc=V./Ns;
% Corriente de Fotogenerada
Isc=5.433;
Alfa=0.037/100;
%variacion de la corriente con la temperatura
Iph=Isc*Radiacion/1000*(1+(Alfa*(Temp-25)));
% Corriente inversa del diodo
Voc_ref=22.2/Ns;
Beta=-0.34/100;
Voc=Voc_ref*(1+(Beta*(Temp-25)));
%for i=1:length(Vc)
%if (Vc(i)>Voc)
%Vc(i)=Voc;
%end
%end
Io=Isc/(exp(Voc/Vt)-1);
Ir=Io;%*(T/298.15)^3*exp(((T/298.15)-1)*1.11*q/(n*K*298.15));

% Funcion a Valuar
I=zeros(size(Vc));
for i=1:50
I = I - (Iph - I - Ir .* ( exp((Vc + I .* Rs) ./ Vt) -1)+(Vc + I .* Rs)/Rp)... 
        ./ (-1 - Ir * (Rs ./ Vt) .* exp((Vc + I .* Rs) ./ Vt)-Rs/Rp); 
end
 end

== matlab function Array/PV panel26/PV module ==
  data: V input; I output; Radiacion input; Temp input
function I = Panel (V,Radiacion,Temp)
% Carga del Electron
q=1.602176e-19;
% Contante de Boltzman
K=1.3806488e-23;
% Constante del material
n=1.3;
% Temperatura en Kelvin
T=273.15+Temp;
% Resistencia serie
Rs=0.015;
% Resistencia Paralelo
Rp=100;
% Calculo del producto de constantes de la exponencial
Vt=(n*K*T)/q;
Ns=36; %celdas en serie.
Vc=V./Ns;
% Corriente de Fotogenerada
Isc=5.433;
Alfa=0.037/100;
%variacion de la corriente con la temperatura
Iph=Isc*Radiacion/1000*(1+(Alfa*(Temp-25)));
% Corriente inversa del diodo
Voc_ref=22.2/Ns;
Beta=-0.34/100;
Voc=Voc_ref*(1+(Beta*(Temp-25)));
%for i=1:length(Vc)
%if (Vc(i)>Voc)
%Vc(i)=Voc;
%end
%end
Io=Isc/(exp(Voc/Vt)-1);
Ir=Io;%*(T/298.15)^3*exp(((T/298.15)-1)*1.11*q/(n*K*298.15));

% Funcion a Valuar
I=zeros(size(Vc));
for i=1:50
I = I - (Iph - I - Ir .* ( exp((Vc + I .* Rs) ./ Vt) -1)+(Vc + I .* Rs)/Rp)... 
        ./ (-1 - Ir * (Rs ./ Vt) .* exp((Vc + I .* Rs) ./ Vt)-Rs/Rp); 
end
 end

== matlab function Array/PV panel27/PV module ==
  data: V input; I output; Radiacion input; Temp input
function I = Panel (V,Radiacion,Temp)
% Carga del Electron
q=1.602176e-19;
% Contante de Boltzman
K=1.3806488e-23;
% Constante del material
n=1.3;
% Temperatura en Kelvin
T=273.15+Temp;
% Resistencia serie
Rs=0.015;
% Resistencia Paralelo
Rp=100;
% Calculo del producto de constantes de la exponencial
Vt=(n*K*T)/q;
Ns=36; %celdas en serie.
Vc=V./Ns;
% Corriente de Fotogenerada
Isc=5.433;
Alfa=0.037/100;
%variacion de la corriente con la temperatura
Iph=Isc*Radiacion/1000*(1+(Alfa*(Temp-25)));
% Corriente inversa del diodo
Voc_ref=22.2/Ns;
Beta=-0.34/100;
Voc=Voc_ref*(1+(Beta*(Temp-25)));
%for i=1:length(Vc)
%if (Vc(i)>Voc)
%Vc(i)=Voc;
%end
%end
Io=Isc/(exp(Voc/Vt)-1);
Ir=Io;%*(T/298.15)^3*exp(((T/298.15)-1)*1.11*q/(n*K*298.15));

% Funcion a Valuar
I=zeros(size(Vc));
for i=1:50
I = I - (Iph - I - Ir .* ( exp((Vc + I .* Rs) ./ Vt) -1)+(Vc + I .* Rs)/Rp)... 
        ./ (-1 - Ir * (Rs ./ Vt) .* exp((Vc + I .* Rs) ./ Vt)-Rs/Rp); 
end
 end

== matlab function Array/PV panel28/PV module ==
  data: V input; I output; Radiacion input; Temp input
function I = Panel (V,Radiacion,Temp)
% Carga del Electron
q=1.602176e-19;
% Contante de Boltzman
K=1.3806488e-23;
% Constante del material
n=1.3;
% Temperatura en Kelvin
T=273.15+Temp;
% Resistencia serie
Rs=0.015;
% Resistencia Paralelo
Rp=100;
% Calculo del producto de constantes de la exponencial
Vt=(n*K*T)/q;
Ns=36; %celdas en serie.
Vc=V./Ns;
% Corriente de Fotogenerada
Isc=5.433;
Alfa=0.037/100;
%variacion de la corriente con la temperatura
Iph=Isc*Radiacion/1000*(1+(Alfa*(Temp-25)));
% Corriente inversa del diodo
Voc_ref=22.2/Ns;
Beta=-0.34/100;
Voc=Voc_ref*(1+(Beta*(Temp-25)));
%for i=1:length(Vc)
%if (Vc(i)>Voc)
%Vc(i)=Voc;
%end
%end
Io=Isc/(exp(Voc/Vt)-1);
Ir=Io;%*(T/298.15)^3*exp(((T/298.15)-1)*1.11*q/(n*K*298.15));

% Funcion a Valuar
I=zeros(size(Vc));
for i=1:50
I = I - (Iph - I - Ir .* ( exp((Vc + I .* Rs) ./ Vt) -1)+(Vc + I .* Rs)/Rp)... 
        ./ (-1 - Ir * (Rs ./ Vt) .* exp((Vc + I .* Rs) ./ Vt)-Rs/Rp); 
end
 end

== matlab function Array/PV panel29/PV module ==
  data: V input; I output; Radiacion input; Temp input
function I = Panel (V,Radiacion,Temp)
% Carga del Electron
q=1.602176e-19;
% Contante de Boltzman
K=1.3806488e-23;
% Constante del material
n=1.3;
% Temperatura en Kelvin
T=273.15+Temp;
% Resistencia serie
Rs=0.015;
% Resistencia Paralelo
Rp=100;
% Calculo del producto de constantes de la exponencial
Vt=(n*K*T)/q;
Ns=36; %celdas en serie.
Vc=V./Ns;
% Corriente de Fotogenerada
Isc=5.433;
Alfa=0.037/100;
%variacion de la corriente con la temperatura
Iph=Isc*Radiacion/1000*(1+(Alfa*(Temp-25)));
% Corriente inversa del diodo
Voc_ref=22.2/Ns;
Beta=-0.34/100;
Voc=Voc_ref*(1+(Beta*(Temp-25)));
%for i=1:length(Vc)
%if (Vc(i)>Voc)
%Vc(i)=Voc;
%end
%end
Io=Isc/(exp(Voc/Vt)-1);
Ir=Io;%*(T/298.15)^3*exp(((T/298.15)-1)*1.11*q/(n*K*298.15));

% Funcion a Valuar
I=zeros(size(Vc));
for i=1:50
I = I - (Iph - I - Ir .* ( exp((Vc + I .* Rs) ./ Vt) -1)+(Vc + I .* Rs)/Rp)... 
        ./ (-1 - Ir * (Rs ./ Vt) .* exp((Vc + I .* Rs) ./ Vt)-Rs/Rp); 
end
 end

== matlab function Array/PV panel30/PV module ==
  data: V input; I output; Radiacion input; Temp input
function I = Panel (V,Radiacion,Temp)
% Carga del Electron
q=1.602176e-19;
% Contante de Boltzman
K=1.3806488e-23;
% Constante del material
n=1.3;
% Temperatura en Kelvin
T=273.15+Temp;
% Resistencia serie
Rs=0.015;
% Resistencia Paralelo
Rp=100;
% Calculo del producto de constantes de la exponencial
Vt=(n*K*T)/q;
Ns=36; %celdas en serie.
Vc=V./Ns;
% Corriente de Fotogenerada
Isc=5.433;
Alfa=0.037/100;
%variacion de la corriente con la temperatura
Iph=Isc*Radiacion/1000*(1+(Alfa*(Temp-25)));
% Corriente inversa del diodo
Voc_ref=22.2/Ns;
Beta=-0.34/100;
Voc=Voc_ref*(1+(Beta*(Temp-25)));
%for i=1:length(Vc)
%if (Vc(i)>Voc)
%Vc(i)=Voc;
%end
%end
Io=Isc/(exp(Voc/Vt)-1);
Ir=Io;%*(T/298.15)^3*exp(((T/298.15)-1)*1.11*q/(n*K*298.15));

% Funcion a Valuar
I=zeros(size(Vc));
for i=1:50
I = I - (Iph - I - Ir .* ( exp((Vc + I .* Rs) ./ Vt) -1)+(Vc + I .* Rs)/Rp)... 
        ./ (-1 - Ir * (Rs ./ Vt) .* exp((Vc + I .* Rs) ./ Vt)-Rs/Rp); 
end
 end

== matlab function Array/PV panel31/PV module ==
  data: V input; I output; Radiacion input; Temp input
function I = Panel (V,Radiacion,Temp)
% Carga del Electron
q=1.602176e-19;
% Contante de Boltzman
K=1.3806488e-23;
% Constante del material
n=1.3;
% Temperatura en Kelvin
T=273.15+Temp;
% Resistencia serie
Rs=0.015;
% Resistencia Paralelo
Rp=100;
% Calculo del producto de constantes de la exponencial
Vt=(n*K*T)/q;
Ns=36; %celdas en serie.
Vc=V./Ns;
% Corriente de Fotogenerada
Isc=5.433;
Alfa=0.037/100;
%variacion de la corriente con la temperatura
Iph=Isc*Radiacion/1000*(1+(Alfa*(Temp-25)));
% Corriente inversa del diodo
Voc_ref=22.2/Ns;
Beta=-0.34/100;
Voc=Voc_ref*(1+(Beta*(Temp-25)));
%for i=1:length(Vc)
%if (Vc(i)>Voc)
%Vc(i)=Voc;
%end
%end
Io=Isc/(exp(Voc/Vt)-1);
Ir=Io;%*(T/298.15)^3*exp(((T/298.15)-1)*1.11*q/(n*K*298.15));

% Funcion a Valuar
I=zeros(size(Vc));
for i=1:50
I = I - (Iph - I - Ir .* ( exp((Vc + I .* Rs) ./ Vt) -1)+(Vc + I .* Rs)/Rp)... 
        ./ (-1 - Ir * (Rs ./ Vt) .* exp((Vc + I .* Rs) ./ Vt)-Rs/Rp); 
end
 end

== matlab function Array/PV panel32/PV module ==
  data: V input; I output; Radiacion input; Temp input
function I = Panel (V,Radiacion,Temp)
% Carga del Electron
q=1.602176e-19;
% Contante de Boltzman
K=1.3806488e-23;
% Constante del material
n=1.3;
% Temperatura en Kelvin
T=273.15+Temp;
% Resistencia serie
Rs=0.015;
% Resistencia Paralelo
Rp=100;
% Calculo del producto de constantes de la exponencial
Vt=(n*K*T)/q;
Ns=36; %celdas en serie.
Vc=V./Ns;
% Corriente de Fotogenerada
Isc=5.433;
Alfa=0.037/100;
%variacion de la corriente con la temperatura
Iph=Isc*Radiacion/1000*(1+(Alfa*(Temp-25)));
% Corriente inversa del diodo
Voc_ref=22.2/Ns;
Beta=-0.34/100;
Voc=Voc_ref*(1+(Beta*(Temp-25)));
%for i=1:length(Vc)
%if (Vc(i)>Voc)
%Vc(i)=Voc;
%end
%end
Io=Isc/(exp(Voc/Vt)-1);
Ir=Io;%*(T/298.15)^3*exp(((T/298.15)-1)*1.11*q/(n*K*298.15));

% Funcion a Valuar
I=zeros(size(Vc));
for i=1:50
I = I - (Iph - I - Ir .* ( exp((Vc + I .* Rs) ./ Vt) -1)+(Vc + I .* Rs)/Rp)... 
        ./ (-1 - Ir * (Rs ./ Vt) .* exp((Vc + I .* Rs) ./ Vt)-Rs/Rp); 
end
 end

== matlab function Array/PV panel33/PV module ==
  data: V input; I output; Radiacion input; Temp input
function I = Panel (V,Radiacion,Temp)
% Carga del Electron
q=1.602176e-19;
% Contante de Boltzman
K=1.3806488e-23;
% Constante del material
n=1.3;
% Temperatura en Kelvin
T=273.15+Temp;
% Resistencia serie
Rs=0.015;
% Resistencia Paralelo
Rp=100;
% Calculo del producto de constantes de la exponencial
Vt=(n*K*T)/q;
Ns=36; %celdas en serie.
Vc=V./Ns;
% Corriente de Fotogenerada
Isc=5.433;
Alfa=0.037/100;
%variacion de la corriente con la temperatura
Iph=Isc*Radiacion/1000*(1+(Alfa*(Temp-25)));
% Corriente inversa del diodo
Voc_ref=22.2/Ns;
Beta=-0.34/100;
Voc=Voc_ref*(1+(Beta*(Temp-25)));
%for i=1:length(Vc)
%if (Vc(i)>Voc)
%Vc(i)=Voc;
%end
%end
Io=Isc/(exp(Voc/Vt)-1);
Ir=Io;%*(T/298.15)^3*exp(((T/298.15)-1)*1.11*q/(n*K*298.15));

% Funcion a Valuar
I=zeros(size(Vc));
for i=1:50
I = I - (Iph - I - Ir .* ( exp((Vc + I .* Rs) ./ Vt) -1)+(Vc + I .* Rs)/Rp)... 
        ./ (-1 - Ir * (Rs ./ Vt) .* exp((Vc + I .* Rs) ./ Vt)-Rs/Rp); 
end
 end

== matlab function Array/PV panel34/PV module ==
  data: V input; I output; Radiacion input; Temp input
function I = Panel (V,Radiacion,Temp)
% Carga del Electron
q=1.602176e-19;
% Contante de Boltzman
K=1.3806488e-23;
% Constante del material
n=1.3;
% Temperatura en Kelvin
T=273.15+Temp;
% Resistencia serie
Rs=0.015;
% Resistencia Paralelo
Rp=100;
% Calculo del producto de constantes de la exponencial
Vt=(n*K*T)/q;
Ns=36; %celdas en serie.
Vc=V./Ns;
% Corriente de Fotogenerada
Isc=5.433;
Alfa=0.037/100;
%variacion de la corriente con la temperatura
Iph=Isc*Radiacion/1000*(1+(Alfa*(Temp-25)));
% Corriente inversa del diodo
Voc_ref=22.2/Ns;
Beta=-0.34/100;
Voc=Voc_ref*(1+(Beta*(Temp-25)));
%for i=1:length(Vc)
%if (Vc(i)>Voc)
%Vc(i)=Voc;
%end
%end
Io=Isc/(exp(Voc/Vt)-1);
Ir=Io;%*(T/298.15)^3*exp(((T/298.15)-1)*1.11*q/(n*K*298.15));

% Funcion a Valuar
I=zeros(size(Vc));
for i=1:50
I = I - (Iph - I - Ir .* ( exp((Vc + I .* Rs) ./ Vt) -1)+(Vc + I .* Rs)/Rp)... 
        ./ (-1 - Ir * (Rs ./ Vt) .* exp((Vc + I .* Rs) ./ Vt)-Rs/Rp); 
end
 end

== matlab function Array/PV panel35/PV module ==
  data: V input; I output; Radiacion input; Temp input
function I = Panel (V,Radiacion,Temp)
% Carga del Electron
q=1.602176e-19;
% Contante de Boltzman
K=1.3806488e-23;
% Constante del material
n=1.3;
% Temperatura en Kelvin
T=273.15+Temp;
% Resistencia serie
Rs=0.015;
% Resistencia Paralelo
Rp=100;
% Calculo del producto de constantes de la exponencial
Vt=(n*K*T)/q;
Ns=36; %celdas en serie.
Vc=V./Ns;
% Corriente de Fotogenerada
Isc=5.433;
Alfa=0.037/100;
%variacion de la corriente con la temperatura
Iph=Isc*Radiacion/1000*(1+(Alfa*(Temp-25)));
% Corriente inversa del diodo
Voc_ref=22.2/Ns;
Beta=-0.34/100;
Voc=Voc_ref*(1+(Beta*(Temp-25)));
%for i=1:length(Vc)
%if (Vc(i)>Voc)
%Vc(i)=Voc;
%end
%end
Io=Isc/(exp(Voc/Vt)-1);
Ir=Io;%*(T/298.15)^3*exp(((T/298.15)-1)*1.11*q/(n*K*298.15));

% Funcion a Valuar
I=zeros(size(Vc));
for i=1:50
I = I - (Iph - I - Ir .* ( exp((Vc + I .* Rs) ./ Vt) -1)+(Vc + I .* Rs)/Rp)... 
        ./ (-1 - Ir * (Rs ./ Vt) .* exp((Vc + I .* Rs) ./ Vt)-Rs/Rp); 
end
 end
